simulink model "ultracap_converter_simplified_PI_control_v5_modified_for_digest"  (R2015a)
settings: Solver=ode45  StartTime=0.0  StopTime=4  FixedStep=TsampleSimulink  MaxStep=1e-6  RelTol=1e-3
values from neighbouring files (symbols this model uses):
  Ea = 4.2622    [me547_based_PI_controller_v3.m]
  Ra = 0.0560    (= 0.056)    [me547_based_PI_controller_v3.m]
  Ts = 1/fs    (= 0.0002)    [load_system_parameters.m]
  Vbat = 48    [load_system_parameters.m]
undefined symbols (not defined in the file or in its folder): fdesignblkfcn, gcbh, ILcommand_z, plecs
libraries: dspsigops x2, dspstat3 x1, simulink x1
settings Model: Creator=Raghav  LastModifiedBy=Anantharaghavan
settings OptimizationCC: ExpressionDepthLimit=2147483647
settings DebuggingCC: UnderspecifiedInitializationDetection=Classic  MergeDetectMultiDrivingBlocksExec=none  SolverPrmCheckMsg=warning  StateNameClashWarn=warning

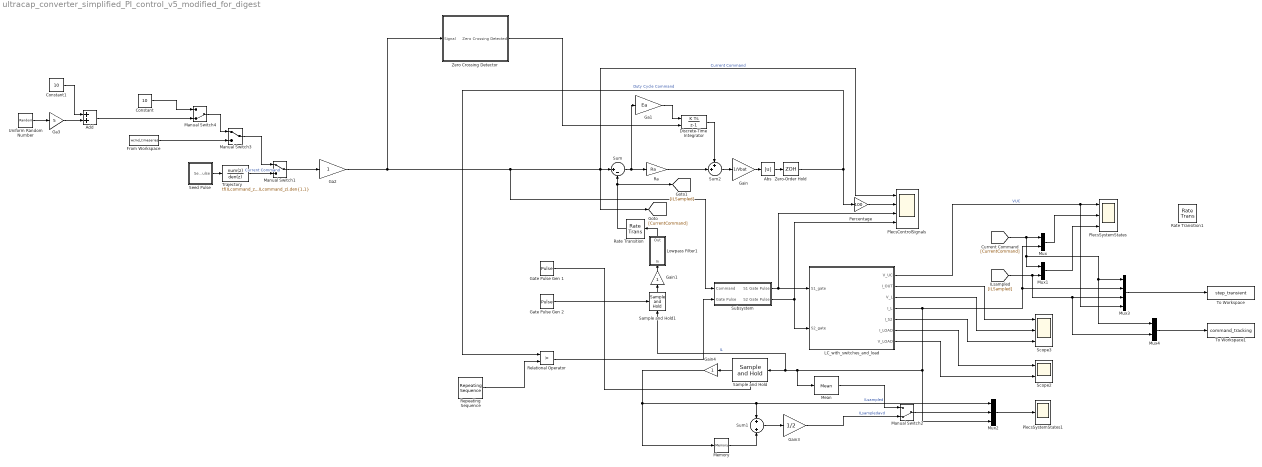
== system ultracap_converter_simplified_PI_control_v5_modified_for_digest ==
  Abs : Abs
  Add : Sum
  Constant : Constant  Value=10
  Constant1 : Constant  Value=10
  Discrete-Time Integrator : DiscreteIntegrator  ExternalReset=rising  InitialConditionSetting=State (most efficient)  SampleTime=Ts
  From Workspace : FromWorkspace  VariableName=wcmd_timeseries  SampleTime=0  Interpolate=off  OutputAfterFinalValue=Holding final value
  Ga1 : Gain  Gain=Ea  SampleTime=Ts
  Ga2 : Gain  SampleTime=Ts
  Ga3 : Gain  Gain=5
  Gain : Gain  Gain=1/Vbat
  Gain1 : Gain  SampleTime=Ts/10
  Gain3 : Gain  Gain=1/2
  Gain4 : Gain  SampleTime=Ts
  Gate Pulse Gen 1 : DiscretePulseGenerator  PulseType=Time based  Period=Ts  PulseWidth=71.42
  Gate Pulse Gen 2 : DiscretePulseGenerator  PulseType=Time based  Period=Ts/10  PulseWidth=71.42
  LC_with_switches_and_load : Subsystem  LoadFcn=plecs('sl', 200);  InitFcn=plecs('sl', 214);  StartFcn=plecs('sl', 208);  StopFcn=plecs('sl', 209);  mask(PlecsCircuit){PLECSData=<binary blob, 2400 chars, not shown>}
      mask prompts: PLECSData "PLECS Data (Do not delete or modify!)"
      mask init:
      | % PLACE CUSTOM INITIALIZATIONS ABOVE
      | % DO NOT REMOVE
      | plecs('sl', 215);
      | % DO NOT REMOVE
      settings: CopyFcn=plecs('sl', 203);  DeleteFcn=plecs('sl', 205);  UndoDeleteFcn=plecs('sl', 206);  PreSaveFcn=plecs('sl', 211);  PostSaveFcn=plecs('sl', 201);  NameChangeFcn=plecs('sl', 210);  DestroyFcn=plecs('sl', 207);  PreCopyFcn=plecs('sl', 216);  OpenFcn=plecs('sl', 202);  ErrorFcn=plerrorfcn
      mask Help: web(['file:///' fullfile(plecsdoc, 'creatingacircuit.html')])
      mask Display: disp('PLECS\nCircuit')
  Lowpass Filter1 : Subsystem  DialogController=fdesignblkfcn  InitFcn=fdesignblkfcn(gcbh, {'InitFcn'});  mask(Lowpass Filter){}
      mask help: Design a lowpass filter
      settings: CopyFcn=fdesignblkfcn(gcbh, {'CopyFcn'});
      mask Help: helpview(mapfilelocation('dsp'), 'dsplowpassfilter');
      mask Display: disp('Lowpass')
  Manual Switch1 : ManualSwitch
  Manual Switch2 : ManualSwitch  CurrentSetting=0
  Manual Switch3 : ManualSwitch
  Manual Switch4 : ManualSwitch  CurrentSetting=0
  Mean : dspstat3/Mean  run=off  reset_popup=None  InputProcessing=Columns as channels (frame based)  directionMode=Each column  dimension=1  treatSBRowAsCol=off  roiEnable=off  roiType=Rectangles  roiPortion=Entire ROI  roiOutput=Individual statistics for each ROI  roiFlag=off  outputDataTypeStr=Inherit: Same as accumulator  outputLastDataTypeStr=Inherit: Same as accumulator  outputMin=[]  outputMax=[]  roundingMode=Floor  overflowMode=off
  Memory : Memory  InheritSampleTime=on  LinearizeMemory=on  LinearizeAsDelay=on
  Mux : Mux  Inputs=2
  Mux1 : Mux  Inputs=2
  Mux2 : Mux  Inputs=3
  Mux3 : Mux
  Mux4 : Mux  Inputs=2
  Percentage : Gain  Gain=100
  PlecsControlSignals : Scope  NumInputPorts=4
      settings: YMin=-5~-6~-1~-1  YMax=-5~-4~1~1  SaveName=PlecsControlSignals
  PlecsSystemStates : Scope  NumInputPorts=3
      settings: ShowLegends=on  TimeRange=1.5  YMin=10~0~3  YMax=10.07~17~15  SaveName=PlecsSystemStates
  PlecsSystemStates1 : Scope
      settings: ShowLegends=on  YMin=0  YMax=10.5  SaveName=PlecsSystemStates1
  Ra : Gain  Gain=Ra  SampleTime=Ts
  Rate Transition : RateTransition  OutPortSampleTime=Ts
  Rate Transition1 : RateTransition
  Relational Operator : RelationalOperator  Priority=50  Operator=>  OutDataTypeStr=boolean
  Repeating Sequence : simulink/Sources/Repeating Sequence  rep_seq_t=[0 Ts]  rep_seq_y=[0 1]
  Sample and Hold : dspsigops/Sample and Hold  trig=Rising edge  initCond=0  latchinput=on
  Sample and Hold1 : dspsigops/Sample and Hold  trig=Rising edge  initCond=0  latchinput=on
  Scope2 : Scope  NumInputPorts=2
      settings: ShowLegends=on  YMin=-5~-5  YMax=5~5  SaveName=ScopeData2
  Scope3 : Scope  NumInputPorts=3
      settings: ShowLegends=on  YMin=0~-50~-5  YMax=3.75~650~5  SaveName=Scope3
  Seed Pulse : Subsystem
  Subsystem : Subsystem
  Sum : Sum  Inputs=|+-
  Sum1 : Sum  Inputs=+|+
  Sum2 : Sum  Inputs=++|
  To Workspace : ToWorkspace  VariableName=step_transient  SaveFormat=Structure With Time  SampleTime=-1
  To Workspace1 : ToWorkspace  VariableName=command_tracking  SaveFormat=Structure With Time  SampleTime=-1
  Trajectory : DiscreteTransferFcn  Numerator=tf(ILcommand_z).num{1,1}  Denominator=tf(ILcommand_z).den{1,1}  SampleTime=Ts
  Uniform Random Number : UniformRandomNumber  SampleTime=Ts
  Zero Crossing Detector : Subsystem
  Zero-Order Hold : ZeroOrderHold  SampleTime=Ts
  wires:
  LC_with_switches_and_load/1(V_UC) -> Mux3/4, PlecsSystemStates/1  "VUC"
  LC_with_switches_and_load/7(V_LOAD) -> Scope2/2
  LC_with_switches_and_load/4(I_L) -> Mux3/2, Mux/2, Mux2/3, Mean/1, Sample and Hold1/1, Sample and Hold/1  "IL"
  LC_with_switches_and_load/6(I_LOAD) -> Scope2/1
  Seed Pulse/1(Seed Pulse) -> Trajectory/1
  Manual Switch1/1 -> Ga2/1
  Sum/1 -> Ga1/1, Ra/1
  Ra/1 -> Sum2/2
  Zero-Order Hold/1 -> Relational Operator/1, Percentage/1  "Duty Cycle Command"
  Repeating Sequence/1 -> Relational Operator/2
  Gain/1 -> Abs/1
  Gate Pulse Gen 1/1 -> Sample and Hold/Trigger
  Memory/1 -> Sum1/2
  Sum1/1 -> Gain3/1
  Mux2/1 -> PlecsSystemStates1/1
  Sample and Hold/1 -> Gain4/1
  Gain4/1 -> Sum1/1, Mux2/1, Memory/1  "ILsampled"
  Gain3/1 -> Manual Switch2/2  "ILsampledavd"
  Mean/1 -> Manual Switch2/1
  Manual Switch2/1 -> Mux2/2
  LC_with_switches_and_load/2(I_OUT) -> Scope3/1
  LC_with_switches_and_load/3(V_L) -> Scope3/2
  LC_with_switches_and_load/5(I_S2) -> Scope3/3
  [CurrentCommand] -> Mux4/1, Mux3/1, Mux1/1, Mux/1
  Mux/1 -> PlecsSystemStates/2
  Mux1/1 -> PlecsSystemStates/3
  [ILSampled] -> Mux4/2, Mux3/3, Mux1/2
  Percentage/1 -> PlecsControlSignals/2
  Sum2/1 -> Gain/1
  Discrete-Time Integrator/1 -> Sum2/1
  Ga1/1 -> Discrete-Time Integrator/1
  Trajectory/1 -> Manual Switch1/2  "Current Command"
  Constant/1 -> Manual Switch4/1
  Lowpass Filter1/1(Out) -> Rate Transition/1
  Sample and Hold1/1 -> Gain1/1
  Gate Pulse Gen 2/1 -> Sample and Hold1/Trigger
  Gain1/1 -> Lowpass Filter1/1(In)
  Rate Transition/1 -> [ILSampled], Sum/2
  Ga2/1 -> Zero Crossing Detector/1(Signal), PlecsControlSignals/1, [CurrentCommand], Sum/1, Subsystem/1(Command)  "Current Command"
  Zero Crossing Detector/1(Zero Crossing Detected) -> Discrete-Time Integrator/2
  Subsystem/2(S2 Gate Pulse) -> LC_with_switches_and_load/2(S2_gate), PlecsControlSignals/4
  Subsystem/1(S1 Gate Pulse) -> PlecsControlSignals/3, LC_with_switches_and_load/1(S1_gate)
  Relational Operator/1 -> Subsystem/2(Gate Pulse)
  Abs/1 -> Zero-Order Hold/1
  Manual Switch3/1 -> Manual Switch1/1
  From Workspace/1 -> Manual Switch3/2
  Manual Switch4/1 -> Manual Switch3/1
  Uniform Random Number/1 -> Ga3/1
  Ga3/1 -> Add/2
  Add/1 -> Manual Switch4/2
  Constant1/1 -> Add/1
  Mux3/1 -> To Workspace/1
  Mux4/1 -> To Workspace1/1

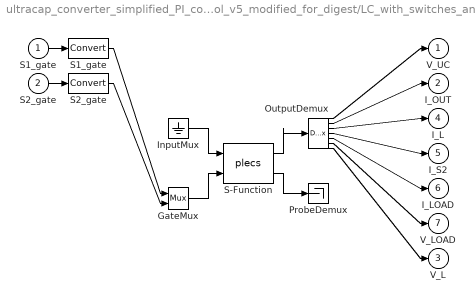
== system ultracap_converter_simplified_PI_control_v5_modified_for_digest/LC_with_switches_and_load ==
  S1_gate : Inport  PortDimensions=1
  S2_gate : Inport  Port=2  PortDimensions=1
  " GateMux " : Mux  Inputs=[ 1 1 ]
  " InputMux " : Ground
  " OutputDemux " : Demux  Outputs=[ 1 1 1 1 1 1 1 ]
  " ProbeDemux " : Terminator
  " S-Function " : S-Function  FunctionName=plecs
  " S1_gate " : DataTypeConversion  SaturateOnIntegerOverflow=on  RndMeth=Zero
  " S2_gate " : DataTypeConversion  SaturateOnIntegerOverflow=on  RndMeth=Zero
  V_UC : Outport  PortDimensions=1
  I_OUT : Outport  Port=2  PortDimensions=1
  V_L : Outport  Port=3  PortDimensions=1
  I_L : Outport  Port=4  PortDimensions=1
  I_S2 : Outport  Port=5  PortDimensions=1
  I_LOAD : Outport  Port=6  PortDimensions=1
  V_LOAD : Outport  Port=7  PortDimensions=1
  wires:
  " S-Function "/2 -> " ProbeDemux "/1
  " GateMux "/1 -> " S-Function "/2
  " InputMux "/1 -> " S-Function "/1
  " S-Function "/1 -> " OutputDemux "/1
  S1_gate/1 -> " S1_gate "/1
  " S1_gate "/1 -> " GateMux "/1
  S2_gate/1 -> " S2_gate "/1
  " S2_gate "/1 -> " GateMux "/2
  " OutputDemux "/1 -> V_UC/1
  " OutputDemux "/2 -> I_OUT/1
  " OutputDemux "/3 -> I_L/1
  " OutputDemux "/4 -> I_S2/1
  " OutputDemux "/5 -> I_LOAD/1
  " OutputDemux "/6 -> V_LOAD/1
  " OutputDemux "/7 -> V_L/1

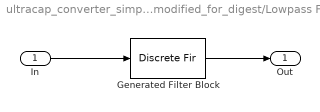
== system ultracap_converter_simplified_PI_control_v5_modified_for_digest/Lowpass Filter1 ==
  In : Inport
  Generated Filter Block : DiscreteFir  Tag=BlockMethodSubSystem  Coefficients=[0.00028387225120272839 -0.00039401751517346924 -0.00051440691195133402 -0.00075899521627578552 -0.0010941645666665207 -0.001504702637592202 -0.0019783528421440035 -0.0024999962120832589 -0.0030483497757197203 -0.0035960077296140168 -0.0041083697578374566 -0.0045449722259692992 -0.0048595556741516856 -0.0050023962125856376 -0.0049212033541305711 -0.0045644105295143556 -0.003882554001486415 -0.0028320966661358892 -0.00137666351787921 0.00050903213237005001 0.0028384532311129655 0.0056092612802152476 0.0088045830229001396 0.012388421653013786 0.016310219840142796 0.020504166250900006 0.024885630758212339 0.029361560221717039 0.033828170940403322 0.038175009739173656 0.04228984466711487 0.046062416914275692 0.049388306387152657 0.05217336678539819 0.054337104315716762 0.055816180296302385 0.056566862063799808 0.056566862063799808 0.055816180296302385 0.054337104315716762 0.05217336678539819 0.049388306387152657 0.046062416914275692 0.04228984466711487 0.038175009739173656 0.033828170940403322 0.029361560221717039 0.024885630758212339 0.020504166250900006 0.016310219840142796 0.012388421653013786 0.0088045830229001396 0.0056092612802152476 0.0028384532311129655 0.00050903213237005001 -0.00137666351787921 -0.0028320966661358892 -0.003882554001486415 -0.0045644105295143556 -0.0049212033541305711 -0.0050023962125856376 -0.0048595556741516856 -0.0045449722259692992 -0.0041083697578374566 -0.0035960077296140168 -0.0030483497757197203 -0.0024999962120832589 -0.0019783528421440035 -0.001504702637592202 -0.0010941645666665207 -0.00075899521627578552 -0.00051440691195133402 -0.00039401751517346924 0.00028387225120272839]  InputProcessing=Columns as channels (frame based)
  Out : Outport
  wires:
  Generated Filter Block/1 -> Out/1
  In/1 -> Generated Filter Block/1

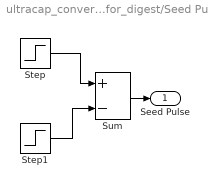
== system ultracap_converter_simplified_PI_control_v5_modified_for_digest/Seed Pulse ==
  Step : Step  Time=10*Ts  SampleTime=0
  Step1 : Step  Time=10*Ts+Ts/2  SampleTime=0
  Sum : Sum  Inputs=+-
  Seed Pulse : Outport
  wires:
  Sum/1 -> Seed Pulse/1
  Step/1 -> Sum/1
  Step1/1 -> Sum/2

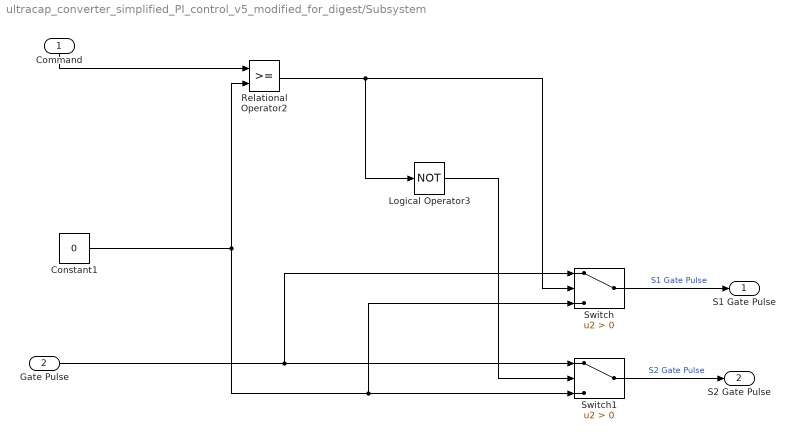
== system ultracap_converter_simplified_PI_control_v5_modified_for_digest/Subsystem ==
  Command : Inport
  Gate Pulse : Inport  Port=2
  Constant1 : Constant  Value=0
  Logical Operator3 : Logic  Operator=NOT  AllPortsSameDT=off  OutDataTypeStr=boolean
  Relational Operator2 : RelationalOperator  OutDataTypeStr=boolean
  Switch : Switch  Criteria=u2 > Threshold
  Switch1 : Switch  Criteria=u2 > Threshold
  S1 Gate Pulse : Outport
  S2 Gate Pulse : Outport  Port=2
  wires:
  Constant1/1 -> Switch1/3, Switch/3, Relational Operator2/2
  Switch1/1 -> S2 Gate Pulse/1  "S2 Gate Pulse"
  Gate Pulse/1 -> Switch1/1, Switch/1
  Switch/1 -> S1 Gate Pulse/1  "S1 Gate Pulse"
  Logical Operator3/1 -> Switch1/2
  Relational Operator2/1 -> Logical Operator3/1, Switch/2
  Command/1 -> Relational Operator2/1

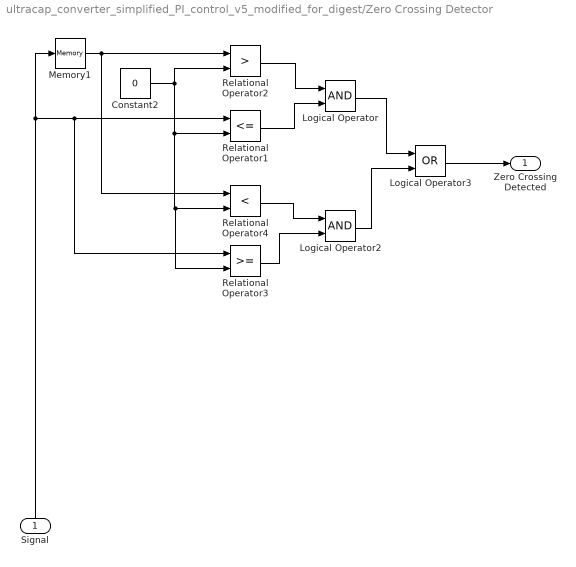
== system ultracap_converter_simplified_PI_control_v5_modified_for_digest/Zero Crossing Detector ==
  Signal : Inport
  Constant2 : Constant  Value=0
  Logical Operator : Logic  AllPortsSameDT=off  OutDataTypeStr=boolean
  Logical Operator2 : Logic  AllPortsSameDT=off  OutDataTypeStr=boolean
  Logical Operator3 : Logic  Operator=OR  AllPortsSameDT=off  OutDataTypeStr=boolean
  Memory1 : Memory  InheritSampleTime=on  LinearizeMemory=on  LinearizeAsDelay=on
  Relational Operator1 : RelationalOperator  Operator=<=  OutDataTypeStr=boolean
  Relational Operator2 : RelationalOperator  Operator=>  OutDataTypeStr=boolean
  Relational Operator3 : RelationalOperator  OutDataTypeStr=boolean
  Relational Operator4 : RelationalOperator  Operator=<  OutDataTypeStr=boolean
  Zero Crossing Detected : Outport
  wires:
  Relational Operator1/1 -> Logical Operator/2
  Logical Operator2/1 -> Logical Operator3/2
  Memory1/1 -> Relational Operator4/1, Relational Operator2/1
  Relational Operator2/1 -> Logical Operator/1
  Constant2/1 -> Relational Operator3/2, Relational Operator4/2, Relational Operator1/2, Relational Operator2/2
  Relational Operator3/1 -> Logical Operator2/2
  Logical Operator/1 -> Logical Operator3/1
  Relational Operator4/1 -> Logical Operator2/1
  Signal/1 -> Relational Operator3/1, Relational Operator1/1, Memory1/1
  Logical Operator3/1 -> Zero Crossing Detected/1
